simulink model "Timing_Synchronizer_Test_Harness"  (R2021b)
settings: Solver=ode3  StartTime=0.0  StopTime=T_Finish  FixedStep=Step_Time  RelTol=1e-3
values from neighbouring files (symbols this model uses):
  Step_Time = 0.01    [Timing_Synchronizer_Schedule.m]    (also in Timing_Synchronizer_Verification.m = median(diff(t)))
settings Model: Creator=salva  LastModifiedBy=salva

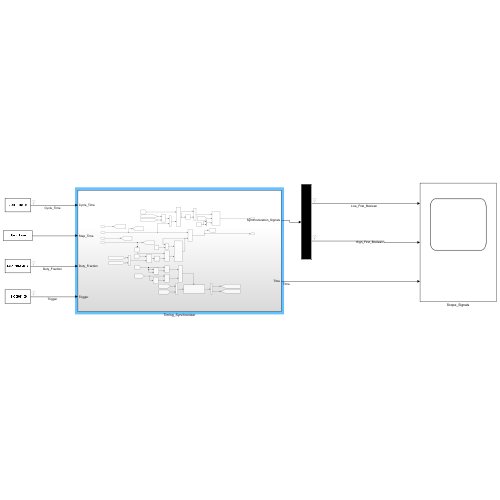
[thumbnail: Simulink's stored preview of the top-level diagram]
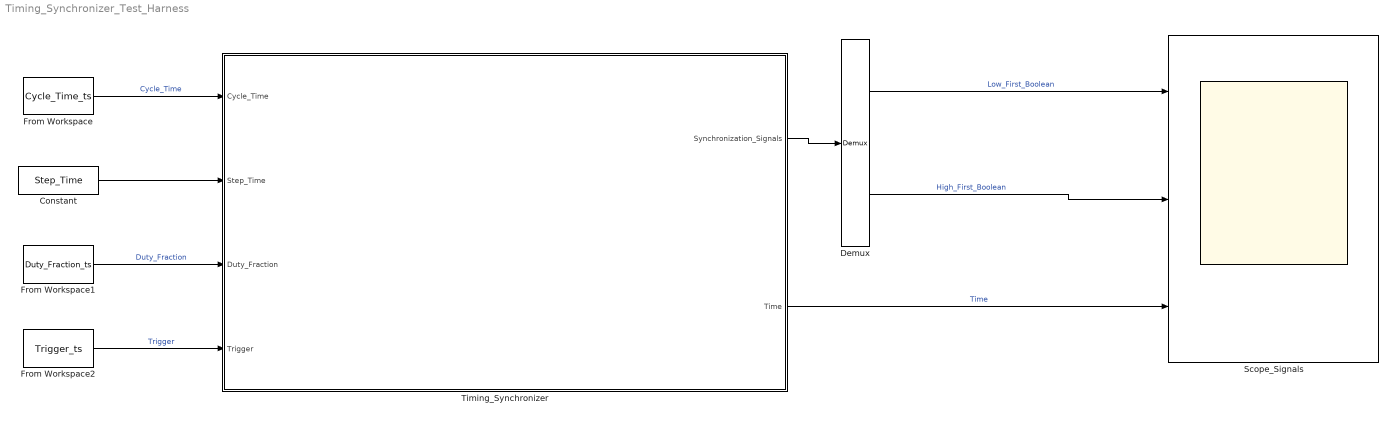
== system Timing_Synchronizer_Test_Harness ==
  Constant : Constant  Value=Step_Time
  Demux : Demux  Outputs=2
  From Workspace : FromWorkspace  VariableName=Cycle_Time_ts
  From Workspace1 : FromWorkspace  VariableName=Duty_Fraction_ts
  From Workspace2 : FromWorkspace  VariableName=Trigger_ts
  Scope_Signals : Scope  NumInputPorts=3
  Timing_Synchronizer : Subsystem
  wires:
  Constant/1 -> Timing_Synchronizer/2(Step_Time)
  From Workspace2/1 -> Timing_Synchronizer/4(Trigger)  "Trigger"
  From Workspace/1 -> Timing_Synchronizer/1(Cycle_Time)  "Cycle_Time"
  Timing_Synchronizer/1(Synchronization_Signals) -> Demux/1
  From Workspace1/1 -> Timing_Synchronizer/3(Duty_Fraction)  "Duty_Fraction"
  Demux/1 -> Scope_Signals/1  "Low_First_Boolean"
  Demux/2 -> Scope_Signals/2  "High_First_Boolean"
  Timing_Synchronizer/2(Time) -> Scope_Signals/3  "Time"

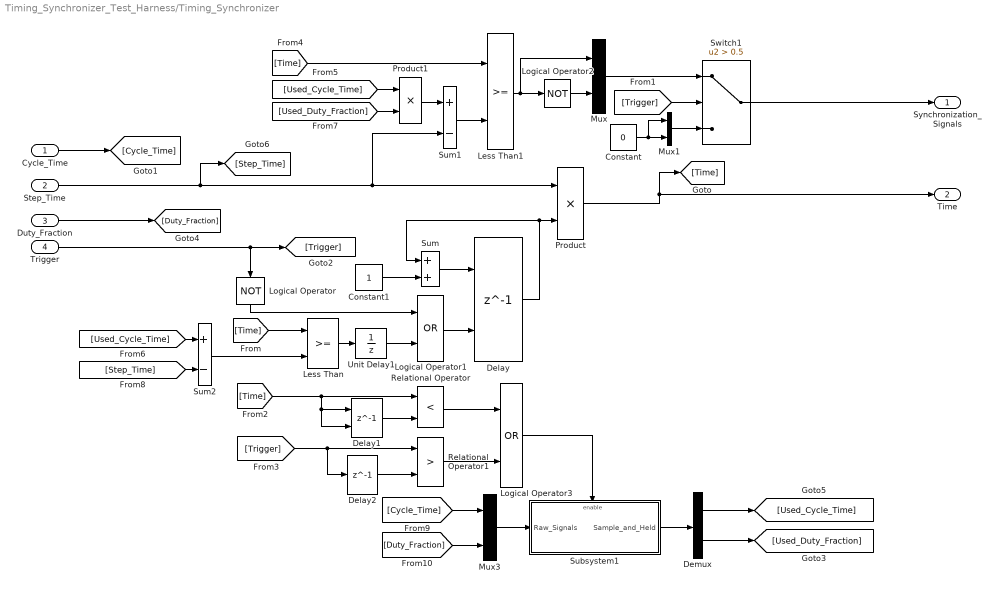
== system Timing_Synchronizer_Test_Harness/Timing_Synchronizer ==
  Cycle_Time : Inport
  Step_Time : Inport  Port=2
  Duty_Fraction : Inport  Port=3
  Trigger : Inport  Port=4
  Constant : Constant  Value=0
  Constant1 : Constant
  Delay : Delay  DelayLength=1  ExternalReset=Level hold
      settings: InputPortMap=u0,r5
  Delay1 : Delay  DelayLength=1  InitialConditionSource=Input port
      settings: InputPortMap=u0,p4
  Delay2 : Delay  DelayLength=1
  Demux : Demux  Outputs=2
  Less Than : RelationalOperator  OutDataTypeStr=boolean  RndMeth=Simplest
  Less Than1 : RelationalOperator  OutDataTypeStr=boolean  RndMeth=Simplest
  Logical Operator : Logic  Operator=NOT  AllPortsSameDT=off  OutDataTypeStr=boolean
  Logical Operator1 : Logic  Operator=OR  AllPortsSameDT=off  OutDataTypeStr=boolean
  Logical Operator2 : Logic  Operator=NOT  AllPortsSameDT=off  OutDataTypeStr=boolean
  Logical Operator3 : Logic  Operator=OR  AllPortsSameDT=off  OutDataTypeStr=boolean
  Mux : Mux  Inputs=2
  Mux1 : Mux  Inputs=2
  Mux3 : Mux  Inputs=2
  Product : Product
  Product1 : Product
  Relational Operator : RelationalOperator  Operator=<  OutDataTypeStr=boolean  RndMeth=Simplest
  Relational Operator1 : RelationalOperator  Operator=>  OutDataTypeStr=boolean  RndMeth=Simplest
  Subsystem1 : Subsystem
  Sum : Sum
  Sum1 : Sum  Inputs=+-
  Sum2 : Sum  Inputs=+-
  Switch1 : Switch  Criteria=u2 > Threshold  Threshold=0.5
  Unit Delay1 : UnitDelay  SampleTime=-1  HasFrameUpgradeWarning=on
  Synchronization_Signals : Outport
  Time : Outport  Port=2
  wires:
  [Used_Cycle_Time] -> Product1/1
  Duty_Fraction/1 -> [Duty_Fraction]
  [Time] -> Less Than1/1
  Unit Delay1/1 -> Logical Operator1/2
  [Time] -> Less Than/1
  Sum/1 -> Delay/1
  Less Than1/1 -> Logical Operator2/1, Mux/1
  Product1/1 -> Sum1/1
  Constant1/1 -> Sum/2
  Delay/1 -> Sum/1, Product/2
  Sum1/1 -> Less Than1/2
  Less Than/1 -> Unit Delay1/1
  Cycle_Time/1 -> [Cycle_Time]
  Logical Operator2/1 -> Mux/2
  Mux/1 -> Switch1/1
  Trigger/1 -> Logical Operator/1, [Trigger]
  Step_Time/1 -> [Step_Time], Sum1/2, Product/1
  Logical Operator1/1 -> Delay/2
  Switch1/1 -> Synchronization_Signals/1
  Constant/1 -> Mux1/1, Mux1/2
  Mux1/1 -> Switch1/3
  [Trigger] -> Switch1/2
  Logical Operator/1 -> Logical Operator1/1
  Product/1 -> Time/1, [Time]
  [Time] -> Delay1/2, Delay1/1, Relational Operator/1
  Delay1/1 -> Relational Operator/2
  Relational Operator/1 -> Logical Operator3/1
  [Trigger] -> Delay2/1, Relational Operator1/1
  Delay2/1 -> Relational Operator1/2
  Relational Operator1/1 -> Logical Operator3/2
  [Cycle_Time] -> Mux3/1
  Mux3/1 -> Subsystem1/1(Raw_Signals)
  [Duty_Fraction] -> Mux3/2
  Subsystem1/1(Sample_and_Held) -> Demux/1
  [Used_Cycle_Time] -> Sum2/1
  [Used_Duty_Fraction] -> Product1/2
  Demux/1 -> [Used_Cycle_Time]
  Demux/2 -> [Used_Duty_Fraction]
  Logical Operator3/1 -> Subsystem1/Enable
  [Step_Time] -> Sum2/2
  Sum2/1 -> Less Than/2

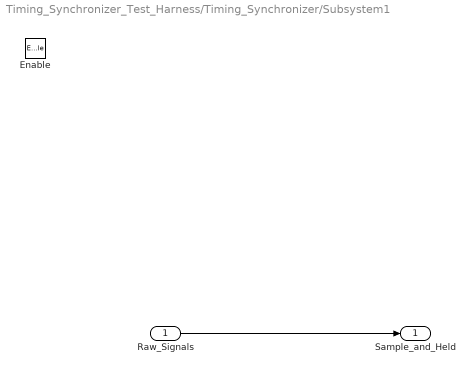
== system Timing_Synchronizer_Test_Harness/Timing_Synchronizer/Subsystem1 ==
  Raw_Signals : Inport
  Enable : EnablePort  StatesWhenEnabling=reset
  Sample_and_Held : Outport
  wires:
  Raw_Signals/1 -> Sample_and_Held/1
